simulink model "MODEL_neural"  (R2024b)
settings: Solver=ode45  StartTime=0.0  StopTime=1  MaxStep=1e-3  RelTol=1e-3  EnableMultiTasking=on
values from neighbouring files (symbols this model uses):
  a = 0.03005    [punkty.m]
  b = -242.5    [punkty.m]
  c = -1.422    [punkty.m]
  d = 0.1096    [punkty.m]
  expected_z = 0.01    [start.m]    (also in start_multi.m = rand*(max_x - 0.002) + 0.001)
  g = 9.81    [punkty.m]
  m = 0.057    [punkty.m]
  R = 4.4    [punkty.m]
undefined symbols (not defined in the file or in its folder): mwag_cal, p_i, p_v, p_z
libraries: simulink x1, rllib x1
settings Model: Creator=Student  LastModifiedBy=agata
settings SolverCC: AlgebraicLoopSolver=TrustRegion
settings DataIOCC: SaveFormat=Array  ReturnWorkspaceOutputs=off
settings OptimizationCC: LifeSpan=inf
settings DebuggingCC: RTPrefix=warning  StringTruncationChecking=none  MaxConsecutiveZCsMsg=warning  MultiTaskDSMMsg=warning  MultiTaskCondExecSysMsg=warning  MultiTaskRateTransMsg=warning  ParameterDowncastMsg=warning  ParameterOverflowMsg=warning  UnconnectedInputMsg=warning  UnconnectedOutputMsg=warning  UnconnectedLineMsg=warning  FrameProcessingCompatibilityMsg=warning  NonCurrentReleaseOperatingPointMsg=warning  SFUnexpectedBacktrackingDiag=warning  SFNoUnconditionalDefaultTransitionDiag=warning  SFOutputUsedAsStateInMooreChartDiag=warning  SFExecutionAtInitializationDiag=none  ArithmeticOperatorsInVariantConditions=warning
settings HardwareCC: ProdBitPerPointer=32  ProdBitPerSizeT=32  ProdBitPerPtrDiffT=32  ProdLargestAtomicFloat=None  ProdIntDivRoundTo=Undefined  ProdEndianess=Unspecified  ProdWordSize=32  ProdHWDeviceType=32-bit Generic
settings ModelReferenceCC: PropagateSignalLabelsOutOfModel=off
settings SFSimCC: SimUseLocalCustomCode=off  CustomCodeUndefinedFunction=UseInterfaceOnly
settings RTWCC: RTWUseLocalCustomCode=off  GPUComputeCapability=3.5
settings CodeAppCC: StateflowObjectComments=on
settings GRTTargetCC: TargetLangStandard=C89/C90 (ANSI)
settings ConfigComp: CovMetricSettings=dw  CovSaveCumulativeToWorkspaceVar=on  CovSaveSingleToWorkspaceVar=on  CovExternalEMLEnable=off

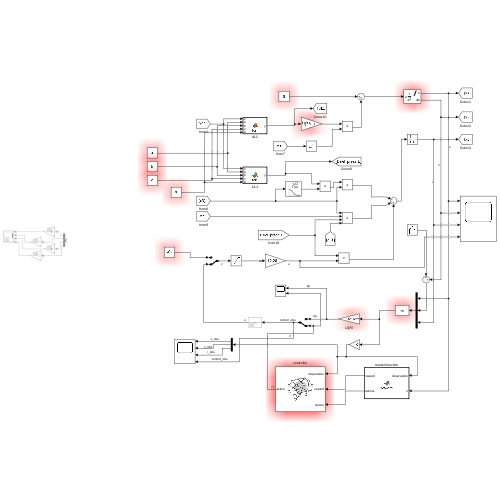
[thumbnail: Simulink's stored preview of the top-level diagram]
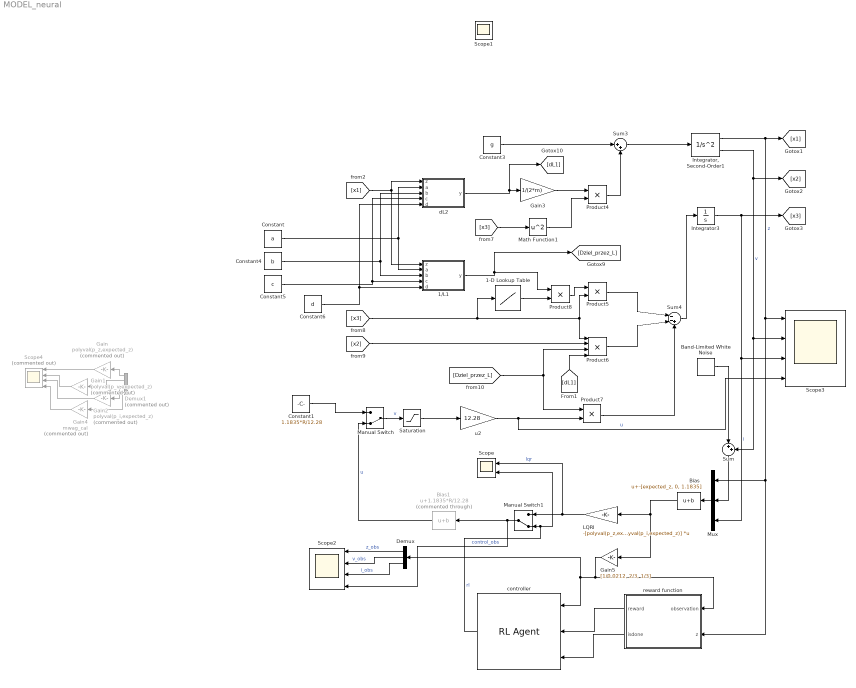
== system MODEL_neural ==
  1-D Lookup Table : Lookup_n-D  NumberOfTableDimensions=1  BreakpointsForDimension1=[0.001 0.63 1.372 2.11 2.828]  Table=[5 4.873015873015873 4.475218658892127 4.364928909952607 4.342291371994342]  InternalRulePriority=Speed  RndMeth=Simplest
  1/L1 : MATLAB Function  TreatAsAtomicUnit=on
  Band-Limited White Noise : simulink/Sources/Band-Limited White Noise  Cov=[0.0001]  Ts=0.005  seed=[23341]
  Bias : Bias  Bias=-[expected_z, 0, 1.1835]  SaturateOnIntegerOverflow=off
  Bias1 : Bias  Commented=through  Bias=1.1835*R/12.28  SaturateOnIntegerOverflow=off
  Constant : Constant  Value=a
  Constant1 : Constant  Value=1.1835*R/12.28
  Constant3 : Constant  Value=g
  Constant4 : Constant  Value=b
  Constant5 : Constant  Value=c
  Constant6 : Constant  Value=d
  Demux : Demux  Outputs=3
  Demux1 : Demux  Commented=on
  Gain : Gain  Commented=on  Gain=polyval(p_z,expected_z)
  Gain1 : Gain  Commented=on  Gain=polyval(p_v,expected_z)
  Gain2 : Gain  Commented=on  Gain=polyval(p_i,expected_z)
  Gain3 : Gain  Gain=1/(2*m)
  Gain4 : Gain  Commented=on  Gain=mwag_cal
  Gain5 : Gain  Gain=[1/0.0212, 2/3, 1/3]
  "Integrator, Second-Order1" : SecondOrderIntegrator  ICX=initial_x  LimitX=on  UpperLimitX=max_x  LowerLimitX=0
  Integrator3 : Integrator  LimitOutput=on  UpperSaturationLimit=999  LowerSaturationLimit=-999  IgnoreLimit=on
  LQRI : Gain  Gain=-[polyval(p_z,expected_z) polyval(p_v,expected_z) polyval(p_i,expected_z)]  Multiplication=Matrix(K*u) (u vector)
  Manual Switch : ManualSwitch  CurrentSetting=0
  Manual Switch1 : ManualSwitch  CurrentSetting=0
  Math Function1 : Math  Operator=square  SignedPower=on
  Mux : Mux  Inputs=3
  Product{4..5,7..8} (4 alike) : Product
  Product6 : Product  Inputs=4
  Saturation : Saturate  UpperLimit=1  LowerLimit=0
  Scope : Scope  NumInputPorts=2
  Scope2 : Scope  NumInputPorts=4
  Scope3 : Scope  NumInputPorts=4
  Scope4 : Scope  Commented=on  NumInputPorts=4
  Sum : Sum  Inputs=|++
  Sum3 : Sum  Inputs=|++
  Sum4 : Sum  Inputs=|--+
  controller : rllib/RL Agent  Agent=agent  ExternalActionAsInput=off  ProvideLastAction=off  ProvideCumRwd=off  TreatAsDirectFeedthrough=on  UseStrictObservationDataTypes=off
  dL2 : MATLAB Function  TreatAsAtomicUnit=on
  reward function : MATLAB Function  TreatAsAtomicUnit=on
  u2 : Gain  Gain=12.28
  Scope1 : Scope
  wires:
  Mux/1 -> Bias/1
  Sum3/1 -> "Integrator, Second-Order1"/1
  1-D Lookup Table/1 -> Product8/2
  [dL1] -> Product6/4
  Gain3/1 -> Product4/1
  Constant6/1 -> 1/L1/5(d), dL2/5(d)
  [x3] -> 1-D Lookup Table/1, Product6/1, Product5/2
  Constant5/1 -> dL2/4(c), 1/L1/4(c)
  Product7/1 -> Sum4/3
  Integrator3/1 -> Mux/3, Scope3/3, [x3]  "i"
  "Integrator, Second-Order1"/1 -> Mux/1, reward function/2(z), Scope3/1, [x1]  "z"
  [x3] -> Math Function1/1
  Sum4/1 -> Integrator3/1
  "Integrator, Second-Order1"/2 -> [x2], Sum/2, Scope3/2  "v"
  Product6/1 -> Sum4/2
  Constant4/1 -> dL2/3(b), 1/L1/3(b)
  Product5/1 -> Sum4/1
  [x1] -> 1/L1/1(z), dL2/1(z)
  Constant3/1 -> Sum3/1
  Product8/1 -> Product5/1
  1/L1/1(y) -> [Dziel_przez_L], Product8/1
  [x2] -> Product6/2
  Constant/1 -> dL2/2(a), 1/L1/2(a)
  dL2/1(y) -> [dL1], Gain3/1
  [Dziel_przez_L] -> Product6/3, Product7/1
  Math Function1/1 -> Product4/2
  Product4/1 -> Sum3/2
  u2/1 -> Scope3/4, Product7/2  "u"
  Saturation/1 -> u2/1
  Constant1/1 -> Manual Switch/1
  Manual Switch/1 -> Saturation/1  "v"
  Manual Switch1/1 -> Bias1/1, Scope2/4  "control_obs"
  reward function/1(reward) -> controller/2
  Demux/1 -> Scope2/1  "z_obs"
  Demux/2 -> Scope2/2  "v_obs"
  Demux/3 -> Scope2/3  "i_obs"
  LQRI/1 -> Scope/1, Manual Switch1/1  "lqr"
  Gain/1 -> Scope4/1
  Gain1/1 -> Scope4/2
  Gain2/1 -> Scope4/3
  Gain4/1 -> Scope4/4
  Demux1/1 -> Gain/1
  Demux1/2 -> Gain1/1
  Demux1/3 -> Gain2/1
  Demux1/4 -> Gain4/1
  Gain5/1 -> reward function/1(observation), controller/1, Demux/1
  Bias1/1 -> Manual Switch/2  "u"
  controller/1 -> Scope/2, Manual Switch1/2  "rl"
  Bias/1 -> Gain5/1, LQRI/1
  reward function/2(isdone) -> controller/3
  Band-Limited White Noise/1 -> Sum/1
  Sum/1 -> Mux/2

== matlab function MODEL_neural/reward function ==
  data: observation input; reward output; isdone output; z input
function [reward,isdone] = reward(observation, z)

% out through the bottom?
hit =(z < 0.002)||(z >=0210);
made_it = abs(observation(1))< 0.005 && abs(observation(2))< 0.005 && abs(observation(3))< 0.005 ;

% calculate reward value
reward = reward_function(observation, made_it, hit);

% done if either failed (crashed) or succeeded
%isdone = (made_it || hit_the_top);
%isdone = made_it;
isdone = 0;

== matlab function MODEL_neural/1//L1 ==
  data: z input; y output; a input; b input; c input; d input
function y = fcn(z,a,b,c,d)
%#codegen
z = max(z, 0);
z = min(z, 30e-3);
y = 1/(a*exp(b*z) + d*exp(c*z));

== matlab function MODEL_neural/dL2 ==
  data: z input; y output; a input; b input; c input; d input
function y = fcn(z,a,b,c,d)
%#codegen
z = max(z, 0);
z = min(z, 30e-3);
%y = - (58297*exp(-(485*z)/2))/8000 - (97407*exp(-(711*z)/500))/625000;
y = a*b*exp(b*z) + c*d*exp(c*z);
